simulink model "Model_SSReducedOrderNominalTrackingSystem"  (R2024b)
settings: Solver=ode45  StartTime=0.0  StopTime=5  RelTol=1e-3
values from neighbouring files (symbols this model uses):
  A_o = A_22 - L_obs*A_12    [Controller_StateSpaceDigitalController.m]
  B_o = [B_2-L_obs*B_1, (A_22-L_obs*A_12)*L_obs + A_21-L_obs*A_11]    [Controller_StateSpaceDigitalController.m]
  C_o = T*[0;1]    [Controller_StateSpaceDigitalController.m]
  D_o = T*[0,1;0,L_obs]    [Controller_StateSpaceDigitalController.m]
settings Model: Creator=Riccardo Grosso  LastModifiedBy=Buton
settings DebuggingCC: AlgebraicLoopMsg=none

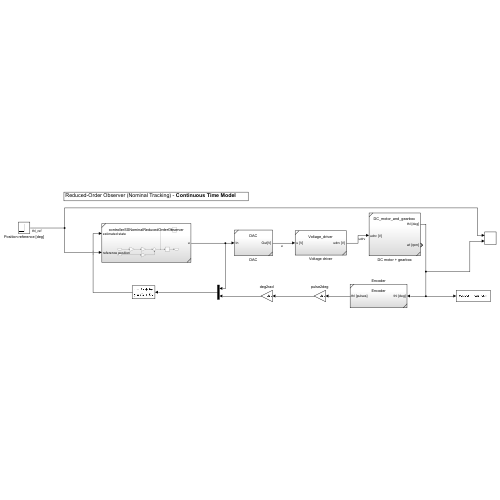
[thumbnail: Simulink's stored preview of the top-level diagram]
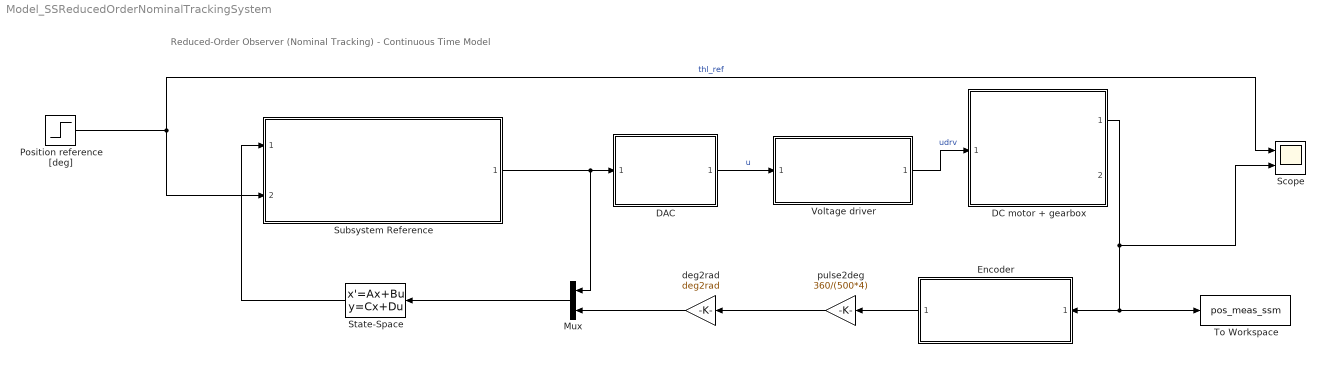
== system Model_SSReducedOrderNominalTrackingSystem ==
  note: Reduced-Order Observer (Nominal Tracking) - Continuous Time Model
  DAC : Subsystem  ReferencedSubsystem=DAC
  DC motor + gearbox : Subsystem  ReferencedSubsystem=DC_motor_and_gearbox
  Encoder : Subsystem  ReferencedSubsystem=Encoder
  Mux : Mux  Inputs=2
  Position reference [deg] : Step  Time=0  After=40  SampleTime=0
  Scope : Scope  NumInputPorts=2
  State-Space : StateSpace  A=A_o  B=B_o  C=C_o  D=D_o  InitialCondition=0
  Subsystem Reference : Subsystem  ReferencedSubsystem=controllerSSNominalReducedOrderObserver
  To Workspace : ToWorkspace  VariableName=pos_meas_ssm  SaveFormat=Timeseries  SampleTime=-1
  Voltage driver : Subsystem  ReferencedSubsystem=Voltage_driver
  deg2rad : Gain  Gain=deg2rad
  pulse2deg : Gain  Gain=360/(500*4)
  wires:
  DAC/1 -> Voltage driver/1  "u"
  Voltage driver/1 -> DC motor + gearbox/1  "udrv"
  Encoder/1 -> pulse2deg/1
  DC motor + gearbox/1 -> Scope/2, To Workspace/1, Encoder/1
  Position reference [deg]/1 -> Subsystem Reference/2, Scope/1  "thl_ref"
  Subsystem Reference/1 -> DAC/1, Mux/1
  pulse2deg/1 -> deg2rad/1
  deg2rad/1 -> Mux/2
  Mux/1 -> State-Space/1
  State-Space/1 -> Subsystem Reference/1
